simulink model "lab_8"  (R2022b)
settings: Solver=FixedStepAuto  StartTime=0.0  StopTime=50  FixedStep=0.01  RelTol=1e-3
values from neighbouring files (symbols this model uses):
  A = [-2 0 0 0 0 1 0 0 0 0 4 -3 ... (16 elements, 4x4)]    [lab_8.mat]    (also in laba9_last.m = [5 -7 -5 1)
  B = [0 2 0 5]    [lab_8.mat]    (also in laba9_last.m = [14;10;6;2])
  C = [1 -1 3 3 ... (first row only)    [laba9_last.m]
settings Model: Creator=osini  LastModifiedBy=osini
settings DebuggingCC: UnconnectedInputMsg=warning  UnconnectedOutputMsg=warning  UnconnectedLineMsg=warning
settings ModelReferenceCC: EnableRefExpFcnMdlSchedulingChecks=on
settings RTWCC: DLArmComputeVersion=19.05

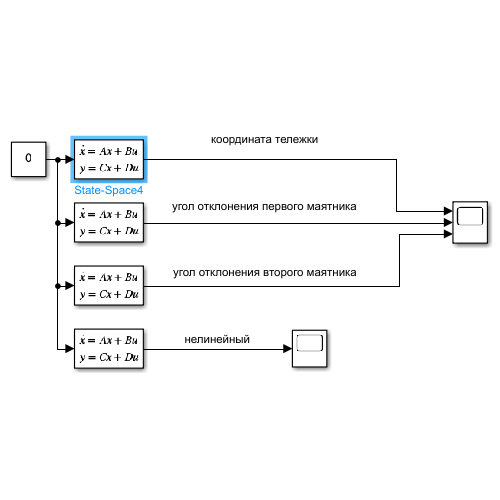
[thumbnail: Simulink's stored preview of the top-level diagram]
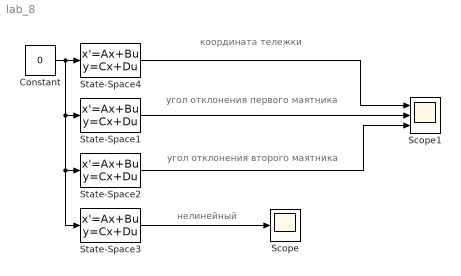
== system lab_8 ==
  note: нелинейный
  note: угол отклонения второго маятника
  note: угол отклонения первого маятника
  note: координата тележки
  Constant : Constant  Value=0
  Scope : Scope
  Scope1 : Scope  NumInputPorts=3
  State-Space1 : StateSpace  A=A  B=[0 0 1 0 0 0]'  C=[0 0 1 0 0 0]  D=zeros(1,1)  InitialCondition=[0.05 0 1 0.1 1 0.15]'
  State-Space2 : StateSpace  A=A  B=[0 0 0 0 1 0]'  C=[0 0 0 0 1 0]  D=zeros(1,1)  InitialCondition=[0.05 0 1 0.1 1 0.15]'
  State-Space3 : StateSpace  A=A  B=B  C=C  D=zeros(3,1)  InitialCondition=[0.05 0 0 0.1 0 0.15]'
  State-Space4 : StateSpace  A=A  B=[1 0 0 0 0 0]'  C=[1 0 0 0 0 0]  D=zeros(1,1)  InitialCondition=[0.05 0 1 0.1 1 0.15]'
  wires:
  State-Space4/1 -> Scope1/1
  Constant/1 -> State-Space1/1, State-Space2/1, State-Space3/1, State-Space4/1
  State-Space1/1 -> Scope1/2
  State-Space2/1 -> Scope1/3
  State-Space3/1 -> Scope/1
